simulink model "LLCv9sim"  (Simulink 7.1)
settings: Solver=ode23  StartTime=0.0  StopTime=0.1  MaxStep=1e-6  RelTol=1e-3
undefined symbols (not defined in the file or in its folder): DiscIntNeverNeededParam
settings Model: Creator=i00184  LastModifiedBy=I00184
settings DebuggingCC: SaveWithParameterizedLinksMsg=none
settings GRTTargetCC: TargetFcnLib=ansi_tfl_tmw.mat

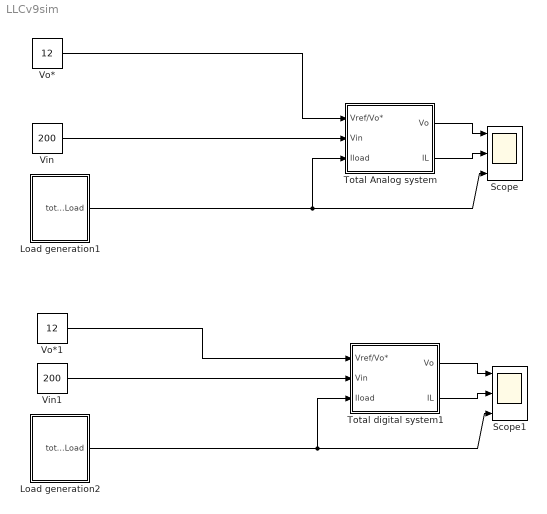
== system LLCv9sim ==
  Load generation1 : Subsystem
  Load generation2 : Subsystem
  Scope : Scope  NumInputPorts=3
      settings: TimeRange=0.001  YMin=12~12.0449~0.73  YMax=12.0001~12.045~0.73
  Scope1 : Scope  NumInputPorts=3
      settings: TimeRange=0.001  YMin=11.87~9.825~0.57  YMax=12.01~10.05~0.63  SaveName=ScopeData2
  Total Analog system : Subsystem
  Total digital system1 : Subsystem
  Vin : Constant  Value=200  OutDataType=sfix(16)  OutScaling=2^0
  Vin1 : Constant  Value=200  OutDataType=sfix(16)  OutScaling=2^0
  Vo* : Constant  Value=12  OutDataType=sfix(16)  OutScaling=2^0
  Vo*1 : Constant  Value=12  OutDataType=sfix(16)  OutScaling=2^0
  wires:
  Load generation1/1(total Load) -> Scope/3, Total Analog system/3(Iload)
  Total Analog system/2(IL) -> Scope/2
  Total Analog system/1(Vo) -> Scope/1
  Vin/1 -> Total Analog system/2(Vin)
  Vo*/1 -> Total Analog system/1(Vref/Vo*)
  Load generation2/1(total Load) -> Scope1/3, Total digital system1/3(Iload)
  Total digital system1/2(IL) -> Scope1/2
  Total digital system1/1(Vo) -> Scope1/1
  Vin1/1 -> Total digital system1/2(Vin)
  Vo*1/1 -> Total digital system1/1(Vref/Vo*)

== system LLCv9sim/Load generation1 ==
  Pulseload : DiscretePulseGenerator  PulseType=Time based  Amplitude=0.5  Period=0.03  PulseWidth=50
  Sum5 : Sum  Inputs=|+++  OutDataType=sfix(16)  OutScaling=2^0
  Transfer Fcn : TransferFcn  Denominator=[1e-6 1]
  loadDC : Constant  Value=0.23  VectorParams1D=off  OutDataType=sfix(16)  OutScaling=2^0
  slew rate1 : RateLimiter  RisingSlewLimit=1/16.67*1e6  FallingSlewLimit=-1/16.67 *1e6  SampleTimeMode=inherited
  total Load : Outport
  wires:
  Transfer Fcn/1 -> slew rate1/1
  Sum5/1 -> Transfer Fcn/1
  slew rate1/1 -> total Load/1
  loadDC/1 -> Sum5/3
  Pulseload/1 -> Sum5/1

== system LLCv9sim/Load generation2 ==
  Pulseload : DiscretePulseGenerator  PulseType=Time based  Amplitude=0.5  Period=0.03  PulseWidth=50
  Sum5 : Sum  Inputs=|+++  OutDataType=sfix(16)  OutScaling=2^0
  Transfer Fcn : TransferFcn  Denominator=[1e-6 1]
  loadDC : Constant  Value=0.1  VectorParams1D=off  OutDataType=sfix(16)  OutScaling=2^0
  slew rate1 : RateLimiter  RisingSlewLimit=0.67/16.67 * 1e6  FallingSlewLimit=-0.67/16.67 *1e6  SampleTimeMode=inherited
  total Load : Outport
  wires:
  Transfer Fcn/1 -> slew rate1/1
  Sum5/1 -> Transfer Fcn/1
  slew rate1/1 -> total Load/1
  loadDC/1 -> Sum5/3
  Pulseload/1 -> Sum5/1

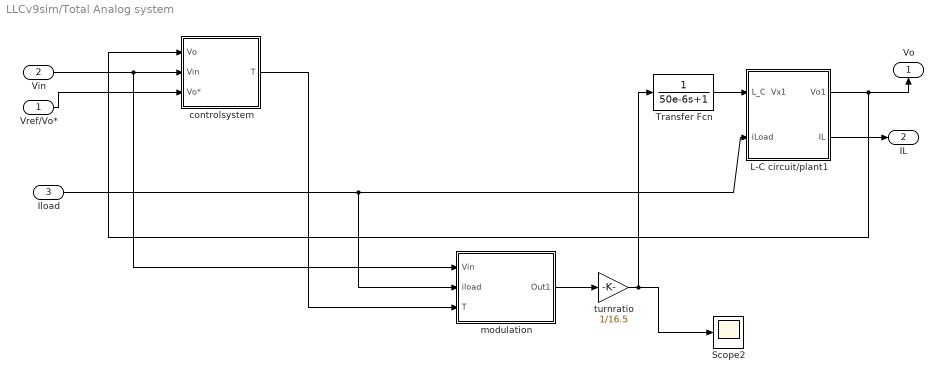
== system LLCv9sim/Total Analog system ==
  Vref/Vo* : Inport
  Vin : Inport  Port=2
  Iload : Inport  Port=3
  L-C circuit/plant1 : Subsystem
  Scope2 : Scope
      settings: YMin=11.546  YMax=11.564  SaveName=ScopeData4
  Transfer Fcn : TransferFcn  Denominator=[50e-6 1]
  controlsystem : Subsystem
  modulation : Subsystem
  turnratio : Gain  Gain=1/16.5  ParameterDataType=sfix(16)  ParameterScaling=2^0  OutDataType=sfix(16)  OutScaling=2^0
  Vo : Outport  Orientation=up
  IL : Outport  Port=2
  wires:
  L-C circuit/plant1/1(Vo1) -> Vo/1, controlsystem/1(Vo)
  Vin/1 -> controlsystem/2(Vin), modulation/1(Vin)
  Vref/Vo*/1 -> controlsystem/3(Vo*)
  L-C circuit/plant1/2(IL) -> IL/1
  Iload/1 -> L-C circuit/plant1/2(iLoad), modulation/2(iload)
  modulation/1(Out1) -> turnratio/1
  turnratio/1 -> Scope2/1, Transfer Fcn/1
  controlsystem/1(T) -> modulation/3(T)
  Transfer Fcn/1 -> L-C circuit/plant1/1(L_C  Vx1)

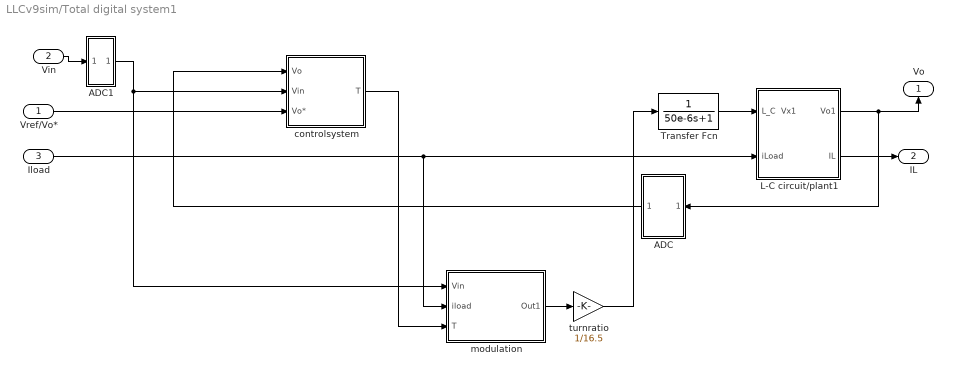
== system LLCv9sim/Total digital system1 ==
  Vref/Vo* : Inport
  Vin : Inport  Port=2
  Iload : Inport  Port=3
  ADC : Subsystem  Orientation=left
  ADC1 : Subsystem
  L-C circuit/plant1 : Subsystem
  Transfer Fcn : TransferFcn  Denominator=[50e-6 1]
  controlsystem : Subsystem
  modulation : Subsystem
  turnratio : Gain  Gain=1/16.5  ParameterDataType=sfix(16)  ParameterScaling=2^0  OutDataType=sfix(16)  OutScaling=2^0
  Vo : Outport  Orientation=up
  IL : Outport  Port=2
  wires:
  L-C circuit/plant1/1(Vo1) -> Vo/1, ADC/1(In1)
  Vin/1 -> ADC1/1(In1)
  Vref/Vo*/1 -> controlsystem/3(Vo*)
  L-C circuit/plant1/2(IL) -> IL/1
  Iload/1 -> L-C circuit/plant1/2(iLoad), modulation/2(iload)
  modulation/1(Out1) -> turnratio/1
  turnratio/1 -> Transfer Fcn/1
  controlsystem/1(T) -> modulation/3(T)
  ADC/1(Out1) -> controlsystem/1(Vo)
  ADC1/1(Out1) -> controlsystem/2(Vin), modulation/1(Vin)
  Transfer Fcn/1 -> L-C circuit/plant1/1(L_C  Vx1)

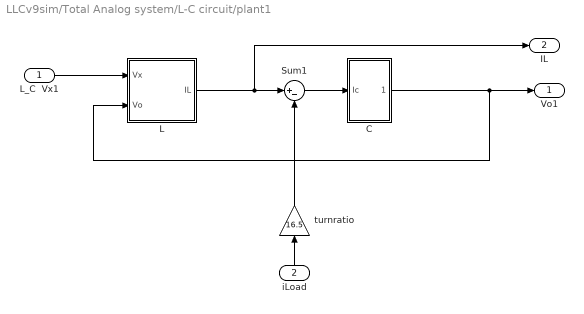
== system LLCv9sim/Total Analog system/L-C circuit/plant1 ==
  L_C  Vx1 : Inport  OutDataType=sfix(16)  OutScaling=2^0
  iLoad : Inport  Orientation=up  Port=2  OutDataType=sfix(16)  OutScaling=2^0
  C : Subsystem
  L : Subsystem
  Sum1 : Sum  Inputs=|+-  OutDataType=sfix(16)  OutScaling=2^0
  turnratio : Gain  Orientation=up  Gain=16.5  ParameterDataType=sfix(16)  ParameterScaling=2^0  OutDataType=sfix(16)  OutScaling=2^0
  Vo1 : Outport  OutDataType=sfix(16)  OutScaling=2^0
  IL : Outport  Port=2  OutDataType=sfix(16)  OutScaling=2^0
  wires:
  iLoad/1 -> turnratio/1
  C/1(Out1) -> Vo1/1, L/2(Vo)
  L_C  Vx1/1 -> L/1(Vx)
  L/1(IL) -> Sum1/1, IL/1
  Sum1/1 -> C/1(Ic)
  turnratio/1 -> Sum1/2

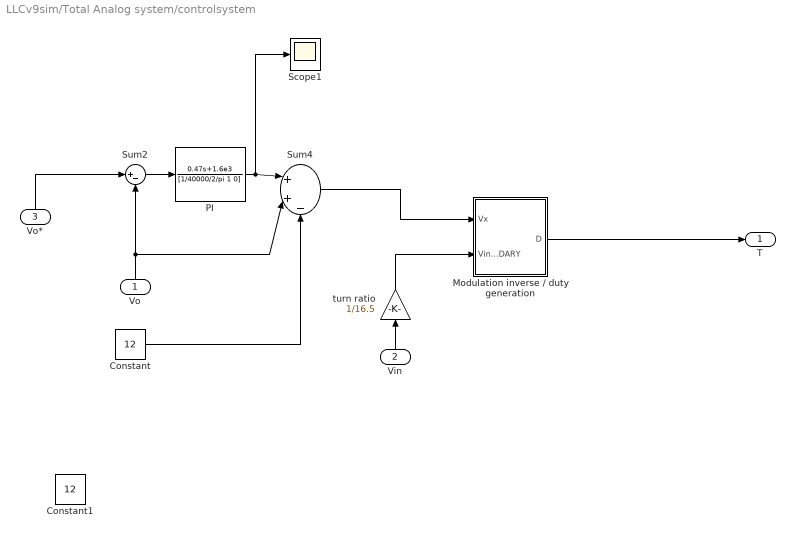
== system LLCv9sim/Total Analog system/controlsystem ==
  Vo : Inport  Orientation=up  OutDataType=sfix(16)  OutScaling=2^0
  Vin : Inport  Orientation=up  Port=2  OutDataType=sfix(16)  OutScaling=2^0
  Vo* : Inport  Orientation=up  Port=3  OutDataType=sfix(16)  OutScaling=2^0
  Constant : Constant  Value=12  OutDataType=sfix(16)  OutScaling=2^0
  Constant1 : Constant  Value=12  OutDataType=sfix(16)  OutScaling=2^0
  Modulation inverse / duty generation : Subsystem
  PI : TransferFcn  Numerator="[0  0.47  1.6e3]"  Denominator=[1/40000/2/pi 1 0]
  Scope1 : Scope
      settings: YMin=-4  YMax=-0.5
  Sum2 : Sum  Inputs=|+-  OutDataType=sfix(16)  OutScaling=2^0
  Sum4 : Sum  Inputs=|++-  OutDataType=sfix(16)  OutScaling=2^0
  turn ratio : Gain  Orientation=up  Gain=1/16.5  ParameterDataType=sfix(16)  ParameterScaling=2^0  OutDataType=sfix(16)  OutScaling=2^0
  T : Outport  OutDataType=sfix(16)  OutScaling=2^0
  wires:
  Vo*/1 -> Sum2/1
  Sum2/1 -> PI/1
  Sum4/1 -> Modulation inverse / duty generation/1(Vx)
  Vin/1 -> turn ratio/1
  Modulation inverse / duty generation/1(D) -> T/1
  Constant/1 -> Sum4/3
  PI/1 -> Sum4/1, Scope1/1
  Vo/1 -> Sum2/2, Sum4/2
  turn ratio/1 -> Modulation inverse / duty generation/2(VinSECONDARY)

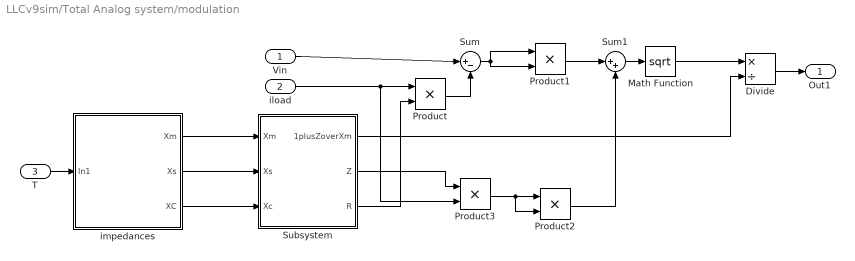
== system LLCv9sim/Total Analog system/modulation ==
  Vin : Inport
  iload : Inport  Port=2
  T : Inport  Port=3
  Divide : Product  Inputs=*/  OutDataType=sfix(16)  OutScaling=2^-10
  Math Function : Math  Operator=sqrt  OutDataType=sfix(16)  OutScaling=2^0  SaturateOnIntegerOverflow=on
  Product{,1..3} (4 alike) : Product  OutDataType=sfix(16)  OutScaling=2^0  RndMeth=Zero
  Subsystem : Subsystem
  Sum : Sum  Inputs=|+-  OutDataType=sfix(16)  OutScaling=2^0
  Sum1 : Sum  Inputs=|++  OutDataType=sfix(16)  OutScaling=2^0
  impedances : Subsystem
  Out1 : Outport
  wires:
  impedances/2(Xs) -> Subsystem/2(Xs)
  impedances/3(XC) -> Subsystem/3(Xc)
  impedances/1(Xm) -> Subsystem/1(Xm)
  Product/1 -> Sum/2
  Subsystem/1(1plusZoverXm) -> Divide/2
  Vin/1 -> Sum/1
  iload/1 -> Product/1, Product3/2
  Divide/1 -> Out1/1
  T/1 -> impedances/1(In1)
  Subsystem/3(R) -> Product/2
  Sum/1 -> Product1/2, Product1/1
  Product1/1 -> Sum1/1
  Product2/1 -> Sum1/2
  Sum1/1 -> Math Function/1
  Product3/1 -> Product2/1, Product2/2
  Subsystem/2(Z) -> Product3/1
  Math Function/1 -> Divide/1

== system LLCv9sim/Total digital system1/ADC ==
  In1 : Inport  Orientation=left
  Quantizer : Quantizer  Orientation=left  QuantizationInterval=14/1024
  Zero-Order Hold : ZeroOrderHold  Orientation=left  SampleTime=1/50000
  Out1 : Outport  Orientation=left
  wires:
  Zero-Order Hold/1 -> Quantizer/1
  Quantizer/1 -> Out1/1
  In1/1 -> Zero-Order Hold/1

== system LLCv9sim/Total digital system1/ADC1 ==
  In1 : Inport  Orientation=left
  Quantizer : Quantizer  Orientation=left  QuantizationInterval=440/1024  LinearizeAsGain=off
  Zero-Order Hold : ZeroOrderHold  Orientation=left  SampleTime=1/100000
  Out1 : Outport  Orientation=left
  wires:
  Zero-Order Hold/1 -> Quantizer/1
  Quantizer/1 -> Out1/1
  In1/1 -> Zero-Order Hold/1

== system LLCv9sim/Total digital system1/L-C circuit/plant1 ==
  L_C  Vx1 : Inport  OutDataType=sfix(16)  OutScaling=2^0
  iLoad : Inport  Orientation=up  Port=2  OutDataType=sfix(16)  OutScaling=2^0
  C : Subsystem
  L : Subsystem
  Sum1 : Sum  Inputs=|+-  OutDataType=sfix(16)  OutScaling=2^0
  turnratio : Gain  Orientation=up  Gain=16.5  ParameterDataType=sfix(16)  ParameterScaling=2^0  OutDataType=sfix(16)  OutScaling=2^0
  Vo1 : Outport  OutDataType=sfix(16)  OutScaling=2^0
  IL : Outport  Port=2  OutDataType=sfix(16)  OutScaling=2^0
  wires:
  iLoad/1 -> turnratio/1
  C/1(Out1) -> Vo1/1, L/2(Vo)
  L_C  Vx1/1 -> L/1(Vx)
  L/1(IL) -> Sum1/1, IL/1
  Sum1/1 -> C/1(Ic)
  turnratio/1 -> Sum1/2

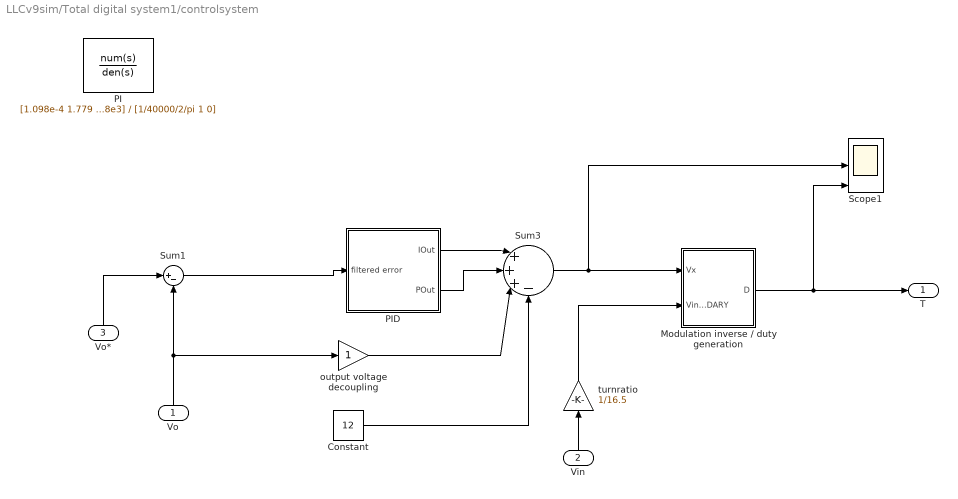
== system LLCv9sim/Total digital system1/controlsystem ==
  Vo : Inport  Orientation=up  OutDataType=sfix(16)  OutScaling=2^0
  Vin : Inport  Orientation=up  Port=2  OutDataType=sfix(16)  OutScaling=2^0
  Vo* : Inport  Orientation=up  Port=3  OutDataType=sfix(16)  OutScaling=2^0
  Constant : Constant  Value=12  OutDataType=sfix(16)  OutScaling=2^0
  Modulation inverse / duty generation : Subsystem
  PI : TransferFcn  Numerator="[1.098e-4 1.779  6.178e3]"  Denominator=[1/40000/2/pi 1 0]
  PID : Subsystem
  Scope1 : Scope  NumInputPorts=3
      settings: TimeRange=0.001  YMin=-1~1.3~4.94e-006  YMax=1~1.5~5.46e-006  SaveName=ScopeData5
  Sum1 : Sum  Inputs=|+-  OutDataType=sfix(16)  OutScaling=2^0
  Sum3 : Sum  Inputs=|+++-  OutDataType=sfix(16)  OutScaling=2^0
  output voltage decoupling : Gain  ParameterDataType=sfix(16)  ParameterScaling=2^0  OutDataType=sfix(16)  OutScaling=2^0
  turnratio : Gain  Orientation=up  Gain=1/16.5  ParameterDataType=sfix(16)  ParameterScaling=2^0  OutDataType=sfix(16)  OutScaling=2^0
  T : Outport  OutDataType=sfix(16)  OutScaling=2^0
  wires:
  Vin/1 -> turnratio/1
  Modulation inverse / duty generation/1(D) -> T/1, Scope1/3
  Sum1/1 -> PID/1(filtered error)
  PID/1(IOut) -> Sum3/1
  Sum3/1 -> Modulation inverse / duty generation/1(Vx), Scope1/2
  Vo/1 -> output voltage decoupling/1, Sum1/2
  Vo*/1 -> Sum1/1
  turnratio/1 -> Modulation inverse / duty generation/2(VinSECONDARY)
  PID/2(POut) -> Sum3/2
  output voltage decoupling/1 -> Sum3/3
  Constant/1 -> Sum3/4

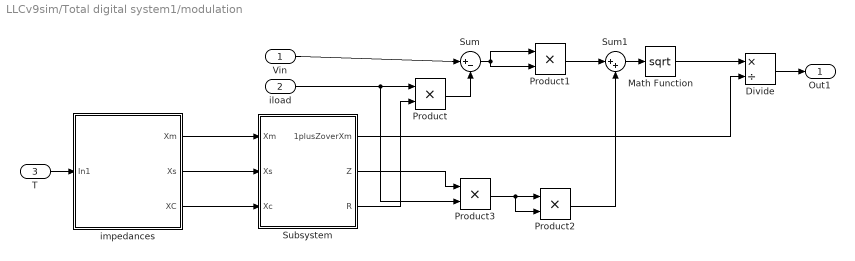
== system LLCv9sim/Total digital system1/modulation ==
  Vin : Inport
  iload : Inport  Port=2
  T : Inport  Port=3
  Divide : Product  Inputs=*/  OutDataType=sfix(16)  OutScaling=2^-10
  Math Function : Math  Operator=sqrt  OutDataType=sfix(16)  OutScaling=2^0  SaturateOnIntegerOverflow=on
  Product{,1..3} (4 alike) : Product  OutDataType=sfix(16)  OutScaling=2^0  RndMeth=Zero
  Subsystem : Subsystem
  Sum : Sum  Inputs=|+-  OutDataType=sfix(16)  OutScaling=2^0
  Sum1 : Sum  Inputs=|++  OutDataType=sfix(16)  OutScaling=2^0
  impedances : Subsystem
  Out1 : Outport
  wires:
  impedances/2(Xs) -> Subsystem/2(Xs)
  impedances/3(XC) -> Subsystem/3(Xc)
  impedances/1(Xm) -> Subsystem/1(Xm)
  Product/1 -> Sum/2
  Subsystem/1(1plusZoverXm) -> Divide/2
  Vin/1 -> Sum/1
  iload/1 -> Product/1, Product3/2
  Divide/1 -> Out1/1
  T/1 -> impedances/1(In1)
  Subsystem/3(R) -> Product/2
  Sum/1 -> Product1/2, Product1/1
  Product1/1 -> Sum1/1
  Product2/1 -> Sum1/2
  Sum1/1 -> Math Function/1
  Product3/1 -> Product2/1, Product2/2
  Subsystem/2(Z) -> Product3/1
  Math Function/1 -> Divide/1

== system LLCv9sim/Total Analog system/L-C circuit/plant1/C ==
  Ic : Inport
  " 1/C" : Gain  Gain=1/360e-6  ParameterDataType=sfix(16)  ParameterScaling=2^0  OutDataType=sfix(16)  OutScaling=2^0
  ESR : Gain  Gain=0.014  ParameterDataType=sfix(16)  ParameterScaling=2^0  OutDataType=sfix(16)  OutScaling=2^0
  Int1 : Integrator  InitialCondition=3.3  LimitOutput=on  LowerSaturationLimit=0
  Sum2 : Sum  Inputs=|++  OutDataType=sfix(16)  OutScaling=2^0
  Out1 : Outport
  wires:
  " 1/C"/1 -> Int1/1
  Ic/1 -> ESR/1, " 1/C"/1
  Int1/1 -> Sum2/1
  Sum2/1 -> Out1/1
  ESR/1 -> Sum2/2

== system LLCv9sim/Total Analog system/L-C circuit/plant1/L ==
  Vx : Inport
  Vo : Inport  Port=2
  Integrator : Integrator  InitialCondition=1  LimitOutput=on  UpperSaturationLimit=200  LowerSaturationLimit=-200
  LSR : Gain  Orientation=left  Gain=0.1  ParameterDataType=sfix(16)  ParameterScaling=2^0  OutDataType=sfix(16)  OutScaling=2^0
  Sum : Sum  Inputs=|+--  OutDataType=sfix(16)  OutScaling=2^0
  prim 1/L : Gain  Gain=1/(4.7e-6)  ParameterDataType=sfix(16)  ParameterScaling=2^0  OutDataType=sfix(16)  OutScaling=2^0
  IL : Outport
  wires:
  Integrator/1 -> IL/1, LSR/1
  Sum/1 -> prim 1/L/1
  prim 1/L/1 -> Integrator/1
  LSR/1 -> Sum/3
  Vo/1 -> Sum/2
  Vx/1 -> Sum/1

== system LLCv9sim/Total Analog system/controlsystem/Modulation inverse / duty generation ==
  Vx : Inport
  VinSECONDARY : Inport  Port=2
  Constant : Constant  Value=5.5E-6  OutDataType=sfix(16)  OutScaling=2^0
  Divide : Product  Inputs=*/  OutDataType=sfix(16)  OutScaling=2^-10
  Saturation : Saturate  UpperLimit=8e-6  LowerLimit=4.54e-6
  Sum : Sum  Inputs=|++  OutDataType=sfix(16)  OutScaling=2^0
  votlagetotimefactor : Gain  Gain=8e-6  ParameterDataType=sfix(16)  ParameterScaling=2^0  OutDataType=sfix(16)  OutScaling=2^0
  D : Outport  OutDataType=sfix(16)  OutScaling=2^0
  wires:
  Vx/1 -> Divide/1
  Saturation/1 -> D/1
  VinSECONDARY/1 -> Divide/2
  Sum/1 -> Saturation/1
  Constant/1 -> Sum/2
  Divide/1 -> votlagetotimefactor/1
  votlagetotimefactor/1 -> Sum/1

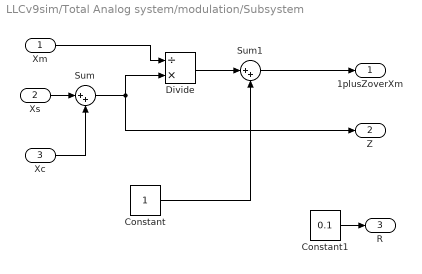
== system LLCv9sim/Total Analog system/modulation/Subsystem ==
  Xm : Inport
  Xs : Inport  Port=2
  Xc : Inport  Port=3
  Constant : Constant  OutDataType=sfix(16)  OutScaling=2^0
  Constant1 : Constant  Value=0.1  OutDataType=sfix(16)  OutScaling=2^0
  Divide : Product  Inputs=/*  OutDataType=sfix(16)  OutScaling=2^-10
  Sum : Sum  Inputs=|++  OutDataType=sfix(16)  OutScaling=2^0
  Sum1 : Sum  Inputs=|++  OutDataType=sfix(16)  OutScaling=2^0
  1plusZoverXm : Outport
  Z : Outport  Port=2
  R : Outport  Port=3
  wires:
  Sum/1 -> Divide/2, Z/1
  Divide/1 -> Sum1/1
  Constant/1 -> Sum1/2
  Xm/1 -> Divide/1
  Sum1/1 -> 1plusZoverXm/1
  Xs/1 -> Sum/1
  Xc/1 -> Sum/2
  Constant1/1 -> R/1

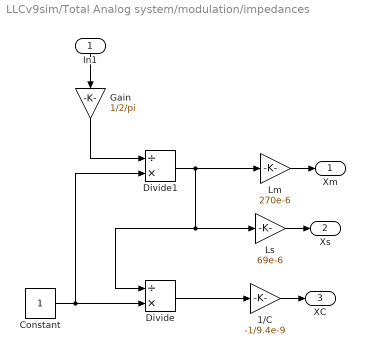
== system LLCv9sim/Total Analog system/modulation/impedances ==
  In1 : Inport  Orientation=down
  1/C : Gain  Gain=-1/9.4e-9  ParameterDataType=sfix(16)  ParameterScaling=2^0  OutDataType=sfix(16)  OutScaling=2^0
  Constant : Constant  OutDataType=sfix(16)  OutScaling=2^0
  Divide : Product  Inputs=/*  OutDataType=sfix(16)  OutScaling=2^-10
  Divide1 : Product  Inputs=/*  OutDataType=sfix(16)  OutScaling=2^-10
  Gain : Gain  Orientation=down  Gain=1/2/pi  ParameterDataType=sfix(16)  ParameterScaling=2^0  OutDataType=sfix(16)  OutScaling=2^0
  Lm : Gain  Gain=270e-6  ParameterDataType=sfix(16)  ParameterScaling=2^0  OutDataType=sfix(16)  OutScaling=2^0
  Ls : Gain  Gain=69e-6  ParameterDataType=sfix(16)  ParameterScaling=2^0  OutDataType=sfix(16)  OutScaling=2^0
  Xm : Outport
  Xs : Outport  Port=2
  XC : Outport  Port=3
  wires:
  Divide/1 -> 1/C/1
  Divide1/1 -> Lm/1, Ls/1, Divide/1
  Constant/1 -> Divide/2, Divide1/2
  Gain/1 -> Divide1/1
  In1/1 -> Gain/1
  Lm/1 -> Xm/1
  Ls/1 -> Xs/1
  1/C/1 -> XC/1

== system LLCv9sim/Total digital system1/L-C circuit/plant1/C ==
  Ic : Inport
  " 1/C" : Gain  Gain=1/360e-6  ParameterDataType=sfix(16)  ParameterScaling=2^0  OutDataType=sfix(16)  OutScaling=2^0
  ESR : Gain  Gain=0.014  ParameterDataType=sfix(16)  ParameterScaling=2^0  OutDataType=sfix(16)  OutScaling=2^0
  Int1 : Integrator  InitialCondition=3.3  LimitOutput=on  LowerSaturationLimit=0
  Sum2 : Sum  Inputs=|++  OutDataType=sfix(16)  OutScaling=2^0
  Out1 : Outport
  wires:
  " 1/C"/1 -> Int1/1
  Ic/1 -> ESR/1, " 1/C"/1
  Int1/1 -> Sum2/1
  Sum2/1 -> Out1/1
  ESR/1 -> Sum2/2

== system LLCv9sim/Total digital system1/L-C circuit/plant1/L ==
  Vx : Inport
  Vo : Inport  Port=2
  Integrator : Integrator  InitialCondition=1  LimitOutput=on  UpperSaturationLimit=200  LowerSaturationLimit=-200
  LSR : Gain  Orientation=left  Gain=0.1  ParameterDataType=sfix(16)  ParameterScaling=2^0  OutDataType=sfix(16)  OutScaling=2^0
  Sum : Sum  Inputs=|+--  OutDataType=sfix(16)  OutScaling=2^0
  prim 1/L : Gain  Gain=1/(4.7e-6)  ParameterDataType=sfix(16)  ParameterScaling=2^0  OutDataType=sfix(16)  OutScaling=2^0
  IL : Outport
  wires:
  Integrator/1 -> IL/1, LSR/1
  Sum/1 -> prim 1/L/1
  prim 1/L/1 -> Integrator/1
  LSR/1 -> Sum/3
  Vo/1 -> Sum/2
  Vx/1 -> Sum/1

== system LLCv9sim/Total digital system1/controlsystem/Modulation inverse / duty generation ==
  Vx : Inport
  VinSECONDARY : Inport  Port=2
  Constant : Constant  Value=5.5e-6  OutDataType=sfix(16)  OutScaling=2^0
  Divide : Product  Inputs=*/  OutDataType=sfix(16)  OutScaling=2^-10
  Saturation : Saturate  UpperLimit=6.67e-6  LowerLimit=4.54e-6
  Sum : Sum  Inputs=|++  OutDataType=sfix(16)  OutScaling=2^0
  voltagetotimefactor : Gain  Gain=8e-6  ParameterDataType=sfix(16)  ParameterScaling=2^0  OutDataType=sfix(16)  OutScaling=2^0
  D : Outport  OutDataType=sfix(16)  OutScaling=2^0
  wires:
  Vx/1 -> Divide/1
  Saturation/1 -> D/1
  VinSECONDARY/1 -> Divide/2
  Sum/1 -> Saturation/1
  Constant/1 -> Sum/2
  Divide/1 -> voltagetotimefactor/1
  voltagetotimefactor/1 -> Sum/1

== system LLCv9sim/Total digital system1/controlsystem/PID ==
  filtered error : Inport
  I : DiscreteIntegrator  gainval=1.6e3  InitialCondition=0.27  SampleTime=1/50000  OutDataType=sfix(16)  OutScaling=2^0  LimitOutput=on  UpperSaturationLimit=12  LowerSaturationLimit=-12  ICPrevOutput=DiscIntNeverNeededParam  ICPrevScaledInput=DiscIntNeverNeededParam
  P : Gain  Gain=0.47  ParameterDataType=sfix(16)  ParameterScaling=2^0  OutDataType=sfix(16)  OutScaling=2^0
  IOut : Outport
  POut : Outport  Port=2
  wires:
  filtered error/1 -> I/1, P/1
  I/1 -> IOut/1
  P/1 -> POut/1

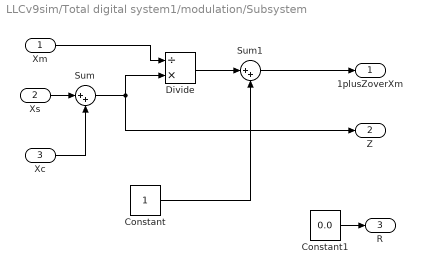
== system LLCv9sim/Total digital system1/modulation/Subsystem ==
  Xm : Inport
  Xs : Inport  Port=2
  Xc : Inport  Port=3
  Constant : Constant  OutDataType=sfix(16)  OutScaling=2^0
  Constant1 : Constant  Value=0.0  OutDataType=sfix(16)  OutScaling=2^0
  Divide : Product  Inputs=/*  OutDataType=sfix(16)  OutScaling=2^-10
  Sum : Sum  Inputs=|++  OutDataType=sfix(16)  OutScaling=2^0
  Sum1 : Sum  Inputs=|++  OutDataType=sfix(16)  OutScaling=2^0
  1plusZoverXm : Outport
  Z : Outport  Port=2
  R : Outport  Port=3
  wires:
  Sum/1 -> Divide/2, Z/1
  Divide/1 -> Sum1/1
  Constant/1 -> Sum1/2
  Xm/1 -> Divide/1
  Sum1/1 -> 1plusZoverXm/1
  Xs/1 -> Sum/1
  Xc/1 -> Sum/2
  Constant1/1 -> R/1

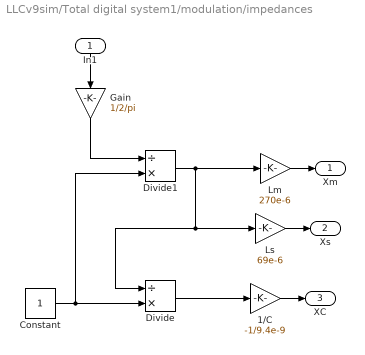
== system LLCv9sim/Total digital system1/modulation/impedances ==
  In1 : Inport  Orientation=down
  1/C : Gain  Gain=-1/9.4e-9  ParameterDataType=sfix(16)  ParameterScaling=2^0  OutDataType=sfix(16)  OutScaling=2^0
  Constant : Constant  OutDataType=sfix(16)  OutScaling=2^0
  Divide : Product  Inputs=/*  OutDataType=sfix(16)  OutScaling=2^-10
  Divide1 : Product  Inputs=/*  OutDataType=sfix(16)  OutScaling=2^-10
  Gain : Gain  Orientation=down  Gain=1/2/pi  ParameterDataType=sfix(16)  ParameterScaling=2^0  OutDataType=sfix(16)  OutScaling=2^0
  Lm : Gain  Gain=270e-6  ParameterDataType=sfix(16)  ParameterScaling=2^0  OutDataType=sfix(16)  OutScaling=2^0
  Ls : Gain  Gain=69e-6  ParameterDataType=sfix(16)  ParameterScaling=2^0  OutDataType=sfix(16)  OutScaling=2^0
  Xm : Outport
  Xs : Outport  Port=2
  XC : Outport  Port=3
  wires:
  Divide/1 -> 1/C/1
  Divide1/1 -> Lm/1, Ls/1, Divide/1
  Constant/1 -> Divide/2, Divide1/2
  Gain/1 -> Divide1/1
  In1/1 -> Gain/1
  Lm/1 -> Xm/1
  Ls/1 -> Xs/1
  1/C/1 -> XC/1
